simulink model "Pitch_control_v5_stop"  (R2017b)
settings: Solver=VariableStepAuto  StartTime=0.0  StopTime=35  MaxStep=0.01  RelTol=1e-3
libraries: simulink x2
settings Model: Creator=robo  LastModifiedBy=ad

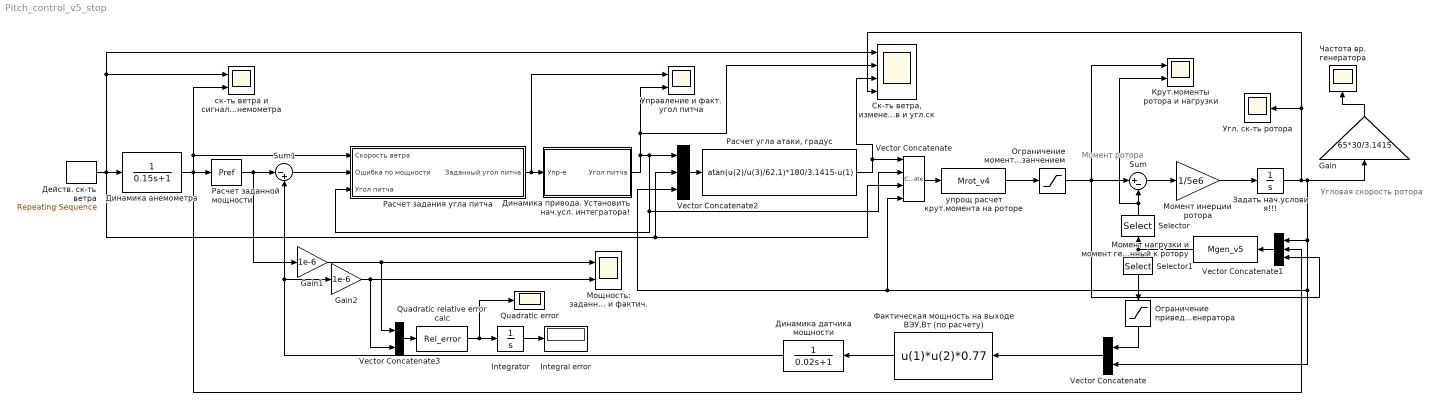
== system Pitch_control_v5_stop ==
  note: Угловая
      | скорость
      | ротора
  note: Момент
      | ротора
  Gain : Gain  Gain=65*30/3.1415
  Gain1 : Gain  Gain=1e-6
  Gain2 : Gain  Gain=1e-6
  Integral error : Display
      settings: Decimation=5
  Integrator : Integrator  ZeroCross=off
  "Quadratic error " : Scope
  Quadratic relative error calc : S-Function  FunctionName=Rel_error  SFunctionDeploymentMode=off  EnableBusSupport=off
  Selector : Selector  InputPortWidth=2  IndexOptions=Index vector (dialog)  Indices=1  OutputSizes=1
  Selector1 : Selector  InputPortWidth=2  IndexOptions=Index vector (dialog)  Indices=2  OutputSizes=1
  Sum : Sum  Inputs=|+-
  Sum1 : Sum  Inputs=|-+
  Vector Concatenate : Concatenate  NumInputs=4
  "Vector Concatenate " : Concatenate
  Vector Concatenate1 : Concatenate  NumInputs=3
  Vector Concatenate2 : Concatenate  NumInputs=3
  Vector Concatenate3 : Concatenate
  "Действ. ск-ть ветра " : simulink/Sources/Repeating Sequence  Description=Входной сигнал по мощности  rep_seq_t=[0 15 21 51]  rep_seq_y=[20 20 26 26]
  Динамика анемометра : TransferFcn  Denominator=[0.15 1]
  Динамика датчика мощности : TransferFcn  Denominator=[0.02 1]
  Динамика привода. Установить нач.усл. интегратора! : Subsystem
  Задать нач.условия!!! : Integrator  InitialCondition=20*6/62.1
  Крут.моменты ротора и нагрузки : Scope  NumInputPorts=2
  Момент инерции ротора : Gain  Gain=1/5e6
  "Момент нагрузки и момент генератора, приведенный к ротору " : S-Function  FunctionName=Mgen_v5  SFunctionDeploymentMode=off  EnableBusSupport=off
  Мощность: заданная и фактич. : Scope  NumInputPorts=2
  Ограничение момента ротора номинальным занчением : Saturate  UpperLimit=5170000  LowerLimit=0
  Ограничение привед.момента генератора : Saturate  UpperLimit=5170000  LowerLimit=0
  Расчет заданной мощности : S-Function  FunctionName=Pref  SFunctionDeploymentMode=off  EnableBusSupport=off
  Расчет задания угла питча : Subsystem
  "Расчет угла атаки, градус" : Fcn  Expr=atan(u(2)/u(3)/62.1)*180/3.1415-u(1)
  "Ск-ть ветра, изменение углов и угл.ск " : Scope  NumInputPorts=4
  Угл. ск-ть ротора : Scope
  "Управление и факт. угол питча " : Scope  NumInputPorts=2
  Фактическая мощность на выходе ВЭУ,Вт (по расчету) : Fcn  Expr=u(1)*u(2)*0.77
  Частота вр. генератора : Scope
  "ск-ть ветра и сигнал анемометра " : Scope  NumInputPorts=2
  упрощ расчет крут.момента на роторе : S-Function  FunctionName=Mrot_v4  SFunctionDeploymentMode=off  EnableBusSupport=off
  wires:
  "Действ. ск-ть ветра "/1 -> "Ск-ть ветра, изменение углов и угл.ск "/1, "ск-ть ветра и сигнал анемометра "/1, Vector Concatenate/3, Vector Concatenate2/2, Динамика анемометра/1
  Расчет заданной мощности/1 -> Sum1/1, Gain1/1
  Vector Concatenate2/1 -> "Расчет угла атаки, градус"/1
  Динамика анемометра/1 -> Vector Concatenate1/2, Расчет заданной мощности/1, "ск-ть ветра и сигнал анемометра "/2, Расчет задания угла питча/1(Скорость ветра)
  Расчет задания угла питча/1(Заданный угол питча) -> "Управление и факт. угол питча "/1, Динамика привода. Установить нач.усл. интегратора!/1(Упр-е)
  Динамика привода. Установить нач.усл. интегратора!/1(Угол питча) -> "Управление и факт. угол питча "/2, "Ск-ть ветра, изменение углов и угл.ск "/2, Vector Concatenate/2, Расчет задания угла питча/3(Угол питча), Vector Concatenate2/1
  "Расчет угла атаки, градус"/1 -> "Ск-ть ветра, изменение углов и угл.ск "/3, Vector Concatenate/1
  Ограничение момента ротора номинальным занчением/1 -> Крут.моменты ротора и нагрузки/1, Vector Concatenate1/3, Sum/1
  Sum/1 -> Момент инерции ротора/1
  Момент инерции ротора/1 -> Задать нач.условия!!!/1
  "Vector Concatenate "/1 -> Фактическая мощность на выходе ВЭУ,Вт (по расчету)/1
  Фактическая мощность на выходе ВЭУ,Вт (по расчету)/1 -> Динамика датчика мощности/1
  Задать нач.условия!!!/1 -> Gain/1, Vector Concatenate1/1, "Vector Concatenate "/2, Vector Concatenate2/3, Vector Concatenate/4, "Ск-ть ветра, изменение углов и угл.ск "/4, Угл. ск-ть ротора/1
  Динамика датчика мощности/1 -> Sum1/2, Gain2/1
  Gain/1 -> Частота вр. генератора/1
  "Момент нагрузки и момент генератора, приведенный к ротору "/1 -> Selector1/1, Selector/1
  Sum1/1 -> Расчет задания угла питча/2(Ошибка по мощности)
  Ограничение привед.момента генератора/1 -> "Vector Concatenate "/1
  Vector Concatenate/1 -> упрощ расчет крут.момента на роторе/1
  упрощ расчет крут.момента на роторе/1 -> Ограничение момента ротора номинальным занчением/1
  Vector Concatenate1/1 -> "Момент нагрузки и момент генератора, приведенный к ротору "/1
  Selector/1 -> Крут.моменты ротора и нагрузки/2, Sum/2
  Selector1/1 -> Ограничение привед.момента генератора/1
  Gain1/1 -> Vector Concatenate3/1, Мощность: заданная и фактич./1
  Gain2/1 -> Vector Concatenate3/2, Мощность: заданная и фактич./2
  Quadratic relative error calc/1 -> Integrator/1, "Quadratic error "/1
  Integrator/1 -> Integral error/1
  Vector Concatenate3/1 -> Quadratic relative error calc/1

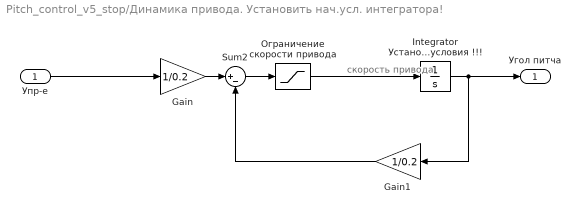
== system Pitch_control_v5_stop/Динамика привода. Установить нач.усл. интегратора! ==
  note: скорость
      |  привода
  Упр-е : Inport
  Gain : Gain  Gain=1/0.2
  Gain1 : Gain  Gain=1/0.2
  Integrator Установить нач.условия !!! : Integrator  InitialCondition=5
  Sum2 : Sum  Inputs=|+-
  Ограничение скорости привода : Saturate  UpperLimit=12  LowerLimit=-12
  Угол питча : Outport
  wires:
  Gain/1 -> Sum2/1
  Ограничение скорости привода/1 -> Integrator Установить нач.условия !!!/1
  Sum2/1 -> Ограничение скорости привода/1
  Gain1/1 -> Sum2/2
  Integrator Установить нач.условия !!!/1 -> Gain1/1, Угол питча/1
  Упр-е/1 -> Gain/1

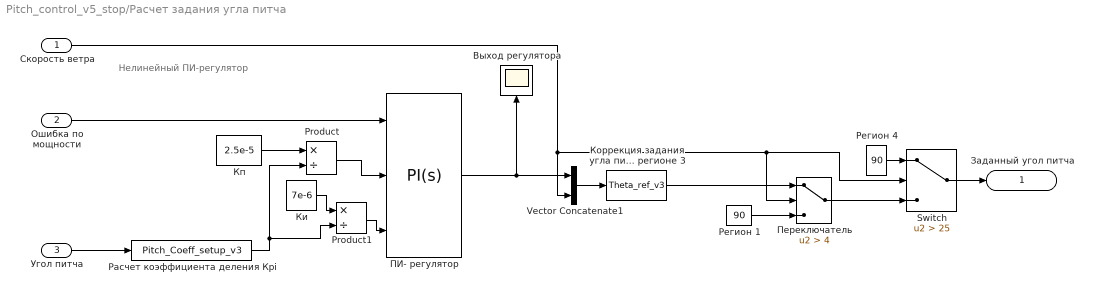
== system Pitch_control_v5_stop/Расчет задания угла питча ==
  note: Нелинейный
      | ПИ-регулятор
  Скорость ветра : Inport
  Ошибка по мощности : Inport  Port=2
  Угол питча : Inport  Port=3
  Product : Product  Inputs=*/
  Product1 : Product  Inputs=*/
  Switch : Switch  Criteria=u2 > Threshold  Threshold=25
  Vector Concatenate1 : Concatenate
  Выход регулятора : Scope
  Ки : Constant  Value=7e-6
  Коррекция задания угла питча с учетом ск-ти ветра в регионе 3 : S-Function  FunctionName=Theta_ref_v3  SFunctionDeploymentMode=off  EnableBusSupport=off
  Кп : Constant  Value=2.5e-5
  ПИ- регулятор : simulink/Continuous/PID Controller  Controller=PI  TimeDomain=Continuous-time  SampleTime=-1  IntegratorMethod=Forward Euler  FilterMethod=Forward Euler  Form=Parallel  UseFilter=on  ControllerParametersSource=external  P=1  I=1  D=0  N=100  InitialConditionSource=internal  InitialConditionForIntegrator=0  InitialConditionForFilter=0  ExternalReset=none  LimitOutput=off  UpperSaturationLimit=inf  LowerSaturationLimit=-inf  LinearizeAsGain=on  AntiWindupMode=none  Kb=1  TrackingMode=off  Kt=1  PParamMin=[]  PParamMax=[]  IParamMin=[]  IParamMax=[]  DParamMin=[]  DParamMax=[]  NParamMin=[]  NParamMax=[]  KbParamMin=[]  KbParamMax=[]  KtParamMin=[]  KtParamMax=[]  POutMin=[]  POutMax=[]  IOutMin=[]  IOutMax=[]  DOutMin=[]  DOutMax=[]  NOutMin=[]  NOutMax=[]  KbOutMin=[]  KbOutMax=[]  KtOutMin=[]  KtOutMax=[]  IntegratorOutMin=[]  IntegratorOutMax=[]  FilterOutMin=[]  FilterOutMax=[]  SumOutMin=[]  SumOutMax=[]  SumI1OutMin=[]  SumI1OutMax=[]  SumI2OutMin=[]  SumI2OutMax=[]  SumI3OutMin=[]  SumI3OutMax=[]  SumDOutMin=[]  SumDOutMax=[]  SaturationOutMin=[]  SaturationOutMax=[]  IntegratorContinuousStateAttributes=''  IntegratorStateMustResolveToSignalObject=off  IntegratorRTWStateStorageClass=Auto  FilterContinuousStateAttributes=''  FilterStateMustResolveToSignalObject=off  FilterRTWStateStorageClass=Auto  DifferentiatorICPrevScaledInput=0  DifferentiatorOutMin=[]  DifferentiatorOutMax=[]  InitialConditionSetting=State (most efficient)  FilterDiffOutCoefMin=[]  FilterDiffOutCoefMax=[]  SumDenOutMin=[]  SumDenOutMax=[]  SumNumOutMin=[]  SumNumOutMax=[]  ReciprocalOutMin=[]  ReciprocalOutMax=[]  DivideOutMin=[]  DivideOutMax=[]  TunerSelectOption=Transfer Function Based (PID Tuner App)
  Переключатель : Switch  Criteria=u2 > Threshold  Threshold=4
  "Расчет коэффициента деления Кpi " : S-Function  FunctionName=Pitch_Coeff_setup_v3  SFunctionDeploymentMode=off  EnableBusSupport=off
  "Регион 1 " : Constant  Value=90
  Регион 4 : Constant  Value=90
  Заданный угол питча : Outport
  wires:
  Угол питча/1 -> "Расчет коэффициента деления Кpi "/1
  Product1/1 -> ПИ- регулятор/3
  "Расчет коэффициента деления Кpi "/1 -> Product/2, Product1/2
  Кп/1 -> Product/1
  Product/1 -> ПИ- регулятор/2
  Ки/1 -> Product1/1
  Ошибка по мощности/1 -> ПИ- регулятор/1
  ПИ- регулятор/1 -> Vector Concatenate1/1, Выход регулятора/1
  Vector Concatenate1/1 -> Коррекция задания угла питча с учетом ск-ти ветра в регионе 3/1
  Переключатель/1 -> Switch/3
  Регион 4/1 -> Switch/1
  Коррекция задания угла питча с учетом ск-ти ветра в регионе 3/1 -> Переключатель/1
  Скорость ветра/1 -> Vector Concatenate1/2, Switch/2, Переключатель/2
  "Регион 1 "/1 -> Переключатель/3
  Switch/1 -> Заданный угол питча/1
